simulink model "SimTest"  (R2016b)
settings: Solver=VariableStepAuto  StartTime=0.0  StopTime=inf  MaxStep=0.001  RelTol=1e-3
libraries: aerolib6dof2 x1, aerolibanim x1, AerialManipulation x1
settings Model: Creator=Administrator  LastModifiedBy=Administrator

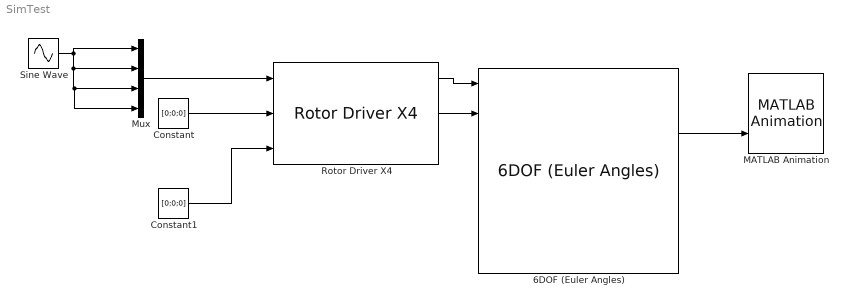
== system SimTest ==
  6DOF (Euler Angles) : aerolib6dof2/6DOF (Euler Angles)  units=Metric (MKS)  mtype=Custom Variable  rep=Euler Angles  xme_0=[0 0 0]  Vm_0=[0 0 0]  eul_0=[0 0 0]  pm_0=[0 0 0]  mass_0=1.0  mass_e=0.5  mass_f=2.0  inertia=eye(3)  inertia_e=eye(3)  inertia_f=2*eye(3)  k_quat=1.0  vre_flag=on
  Constant : Constant  Value=[0;0;0]
  Constant1 : Constant  Value=[0;0;0]
  MATLAB Animation : aerolibanim/MATLAB Animation  Tag=Matlab Animation 6 DOF  Vehicles=1  Geometries='astredwedge.mat'  BoundingBoxCoordinates=[-50,50,-50,50,-50,50]  CameraOffset=[-100,-50,-10]  CameraViewAngle=2.0  SampleTime=0.2  FigurePosition=[403,157,559,360]
  Mux : Mux
  Rotor Driver X4 : AerialManipulation/Rotor Driver X4  l=0.18  Fe=[ [0;0;1],[0;0;1],[0;0;1],[0;0;1] ]  r=[ [0.18;0;0],[0;0.18;0],[-0.18;0;0],[0;-0.18;0] ]  Td=[ [0;0;1], [0;0;-1],[0;0;1],[0;0;-1] ]  Kct=3.16e-05  Ktf=0.01
  Sine Wave : Sin  Amplitude=100  SampleTime=0
  wires:
  Rotor Driver X4/1 -> 6DOF (Euler Angles)/1
  Rotor Driver X4/2 -> 6DOF (Euler Angles)/2
  6DOF (Euler Angles)/3 -> MATLAB Animation/2
  Constant/1 -> Rotor Driver X4/2
  Constant1/1 -> Rotor Driver X4/3
  Sine Wave/1 -> Mux/1, Mux/4, Mux/3, Mux/2
  Mux/1 -> Rotor Driver X4/1
